simulink model "model_siso"  (Simulink 7.4)
settings: Solver=ode3  StartTime=0.0  StopTime=T-Ts  FixedStep=Ts  RelTol=1e-3
values from neighbouring files (symbols this model uses):
  sys = sys(1:2,1:2)    [main_mimo.m]    (also in main_siso.m = sys(1,2))
  Ts = 1/Fs    [definitions.m]    (also in main_hess.m = 0.05; main_mimo.m = 0.1; main_rider.m = 0.02; main_rider_time.m = 0.02)
libraries: cstblocks x1
settings Model: Creator=Peter  LastModifiedBy=Peter
settings DataIOCC: SaveOutput=off  SaveTime=off

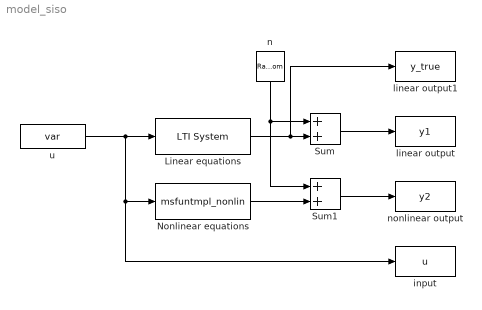
== system model_siso ==
  Linear equations : cstblocks/LTI System  SystemSampleTime=-1  sys=sys;  IC=zeros(4,1);
  Nonlinear equations : M-S-Function  FunctionName=msfuntmpl_nonlin
  Sum : Sum  OutDataType=sfix(16)  OutScaling=2^0  SaturateOnIntegerOverflow=on  InputSameDT=on  OutDataTypeStr=Inherit: Same as first input
  Sum1 : Sum  OutDataType=sfix(16)  OutScaling=2^0  SaturateOnIntegerOverflow=on  InputSameDT=on  OutDataTypeStr=Inherit: Same as first input
  input : ToWorkspace  VariableName=u  SampleTime=Ts  SaveFormat=Structure With Time
      settings: Description=output
  linear output : ToWorkspace  VariableName=y1  SampleTime=Ts  SaveFormat=Structure With Time
      settings: Description=output
  linear output1 : ToWorkspace  VariableName=y_true  SampleTime=Ts  SaveFormat=Structure With Time
      settings: Description=output
  n : RandomNumber  Variance=0.0001  Seed=61  SampleTime=Ts
  nonlinear output : ToWorkspace  VariableName=y2  SampleTime=Ts  SaveFormat=Structure With Time
      settings: Description=output
  u : FromWorkspace  VariableName=var  SampleTime=Ts  Interpolate=off  OutputAfterFinalValue=Setting to zero
  wires:
  Linear equations/1 -> Sum/2, linear output1/1
  n/1 -> Sum/1, Sum1/1
  Sum/1 -> linear output/1
  u/1 -> Linear equations/1, input/1, Nonlinear equations/1
  Nonlinear equations/1 -> Sum1/2
  Sum1/1 -> nonlinear output/1
